simulink model "SecRwRtStFwdBkwdTrgtPosSelc"  (R2018b)
settings: Solver=FixedStepDiscrete  StartTime=0.0  StopTime=10.0  FixedStep=0.01  RelTol=1e-3
undefined symbols (not defined in the file or in its folder): KeSMSw4SAcsMd23SecRwRtStFrwdBkwdPos_Val, KeSMSw4SAcsMd23SecRwRtStFrwdBkwdPosMax_Val, KeSMSw4SAcsMd23SecRwRtStFrwdBkwdPosMin_Val, KeSMSw4SAcsMd24SecRwRtStFrwdBkwdPos_Val, KeSMSw4SAcsMd24SecRwRtStFrwdBkwdPosMax_Val, KeSMSw4SAcsMd24SecRwRtStFrwdBkwdPosMin_Val, KeSMSw4SAcsMd25SecRwRtStFrwdBkwdPos_Val, KeSMSw4SAcsMd25SecRwRtStFrwdBkwdPosMax_Val, KeSMSw4SAcsMd25SecRwRtStFrwdBkwdPosMin_Val, KeSMSw4SAcsMd26SecRwRtStFrwdBkwdPos_Val, KeSMSw4SAcsMd26SecRwRtStFrwdBkwdPosMax_Val, KeSMSw4SAcsMd26SecRwRtStFrwdBkwdPosMin_Val, KeSMSw4SLegrstOpenMdSecRwRtStFrwdBkwdPos_Val, KeSMSw4SLegrstOpenMdSecRwRtStFrwdBkwdPosMax_Val, KeSMSw4SLegrstOpenMdSecRwRtStFrwdBkwdPosMin_Val, KeSMSw4SLyingMDSecRwRtStFrwdBkwdPos_Val, KeSMSw4SLyingMDSecRwRtStFrwdBkwdPosMax_Val, KeSMSw4SLyingMDSecRwRtStFrwdBkwdPosMin_Val, KeSMSw4SVIPMDSecRwRtStFrwdBkwdPos_Val, KeSMSw4SVIPMDSecRwRtStFrwdBkwdPosMax_Val, KeSMSw4SVIPMDSecRwRtStFrwdBkwdPosMin_Val, KeSMSw6sAcsEntrySecRwRtStFrwdBkwdPos_Val, KeSMSw6sAcsEntrySecRwRtStFrwdBkwdPosMax_Val, KeSMSw6sAcsEntrySecRwRtStFrwdBkwdPosMin_Val, KeSMSw6sAcsExtSecRwRtStFrwdBkwdPos_Val, KeSMSw6sAcsExtSecRwRtStFrwdBkwdPosMax_Val, KeSMSw6sAcsExtSecRwRtStFrwdBkwdPosMin_Val, KeSMSw6sFamilyMdSecRwRtStFrwdBkwdPos_Val, KeSMSw6sFamilyMdSecRwRtStFrwdBkwdPosMax_Val, KeSMSw6sFamilyMdSecRwRtStFrwdBkwdPosMin_Val, KeSMSw6sFamilyRMdSecRwRtStFrwdBkwdPos_Val, KeSMSw6sFamilyRMdSecRwRtStFrwdBkwdPosMax_Val, KeSMSw6sFamilyRMdSecRwRtStFrwdBkwdPosMin_Val, KeSMSw6sVIPSecRwRtStFrwdBkwdPos_Val, KeSMSw6sVIPSecRwRtStFrwdBkwdPosMax_Val, KeSMSw6sVIPSecRwRtStFrwdBkwdPosMin_Val, KeSMSwAcsEntrySecRwRtStFrwdBkwdPos_Val, KeSMSwAcsEntrySecRwRtStFrwdBkwdPosMax_Val, KeSMSwAcsEntrySecRwRtStFrwdBkwdPosMin_Val, KeSMSwAcsExtSecRwRtStFrwdBkwdPos_Val, KeSMSwAcsExtSecRwRtStFrwdBkwdPosMax_Val, KeSMSwAcsExtSecRwRtStFrwdBkwdPosMin_Val, KeSMSwAcsMd8SecRwRtStFrwdBkwdPos_Val, KeSMSwAcsMd8SecRwRtStFrwdBkwdPosMax_Val, KeSMSwAcsMd8SecRwRtStFrwdBkwdPosMin_Val, KeSMSwAcsMd9SecRwRtStFrwdBkwdPos_Val, KeSMSwAcsMd9SecRwRtStFrwdBkwdPosMax_Val, KeSMSwAcsMd9SecRwRtStFrwdBkwdPosMin_Val, KeSMSwFamilyMdSecRwRtStFrwdBkwdPos_Val, KeSMSwFamilyMdSecRwRtStFrwdBkwdPosMax_Val, KeSMSwFamilyMdSecRwRtStFrwdBkwdPosMin_Val, KeSMSwFamilyRMdSecRwRtStFrwdBkwdPos_Val, KeSMSwFamilyRMdSecRwRtStFrwdBkwdPosMax_Val, KeSMSwFamilyRMdSecRwRtStFrwdBkwdPosMin_Val, KeSMSwVIPSecRwRtStFrwdBkwdPos_Val, KeSMSwVIPSecRwRtStFrwdBkwdPosMax_Val, KeSMSwVIPSecRwRtStFrwdBkwdPosMin_Val
libraries: TrgtPosSelcLib x16
settings Model: Creator=sn2xws  LastModifiedBy=sn2xws
settings Model: ModifiedHistory=|
  | 2023.8.1 V2.0.0 CR401790 增加模式21-26
  | Issue 566045 全躺，vip，腿托打开增加前后位置
  | 2024.7.9 V3.0.0 557模式流程V1.9
settings DataIOCC: SaveFormat=StructureWithTime
settings OptimizationCC: DefaultParameterBehavior=Inlined  EnhancedBackFolding=on  PassReuseOutputArgsAs=Individual arguments  ZeroExternalMemoryAtStartup=off  ZeroInternalMemoryAtStartup=off  OptimizeBlockOrder=speed  DifferentSizesBufferReuse=on  OptimizationCustomize=off
settings DebuggingCC: ParameterTunabilityLossMsg=error
settings ModelReferenceCC: ModelReferenceNumInstancesAllowed=Single
settings SFSimCC: MATLABDynamicMemAlloc=off
settings RTWCC: SystemTargetFile=autosar.tlc  GenCodeOnly=on  TemplateMakefile=ert_default_tmf  Description=AUTOSAR  GenerateReport=on  IncludeHyperlinkInReport=on  LaunchReport=on  GenerateTraceInfo=on  GenerateTraceReport=on  GenerateTraceReportSl=on  GenerateTraceReportSf=on  GenerateTraceReportEml=on
settings CodeAppCC: ForceParamTrailComments=on  IgnoreCustomStorageClasses=off  OperatorAnnotations=on  SimulinkDataObjDesc=on  SFDataObjDesc=on  InsertBlockDesc=on
settings STFCustomTargetCC: TargetLangStandard=C99 (ISO)  MultiwordLength=256  ParMdlRefBuildCompliant=on  CompOptLevelCompliant=on  IncludeMdlTerminateFcn=off  CombineOutputUpdateFcns=on  SuppressErrorStatus=on  ERTCustomFileBanners=on  SupportNonFinite=off  SupportComplex=off  SupportContinuousTime=off  SupportNonInlinedSFcns=off  RemoveResetFunc=on  MATLABClassNameForMDSCustomization=Simulink.SoftwareTarget.ERTCustomization  AutosarCompliant=on  UseToolchainInfoCompliant=on  LookupTableObjectStructAxisOrder=2,1,3,4,...  LUTObjectStructOrderEvenSpacing=Size,Table,Breakpoints  SystemTargetFile=autosar.tlc
settings ERTTargetCC: TargetLangStandard=C99 (ISO)  ConcurrentExecutionCompliant=off  IncludeMdlTerminateFcn=off  SuppressErrorStatus=on  SupportNonFinite=off  SupportComplex=off  ModelStepFunctionPrototypeControlCompliant=off  CPPClassGenCompliant=off  AutosarCompliant=on  LookupTableObjectStructAxisOrder=2,1,3,4,...  LUTObjectStructOrderEvenSpacing=Size,Table,Breakpoints  InlinedParameterPlacement=NonHierarchical  ERTCustomFileTemplate=example_file_process.tlc  ERTFilePackagingFormat=Compact

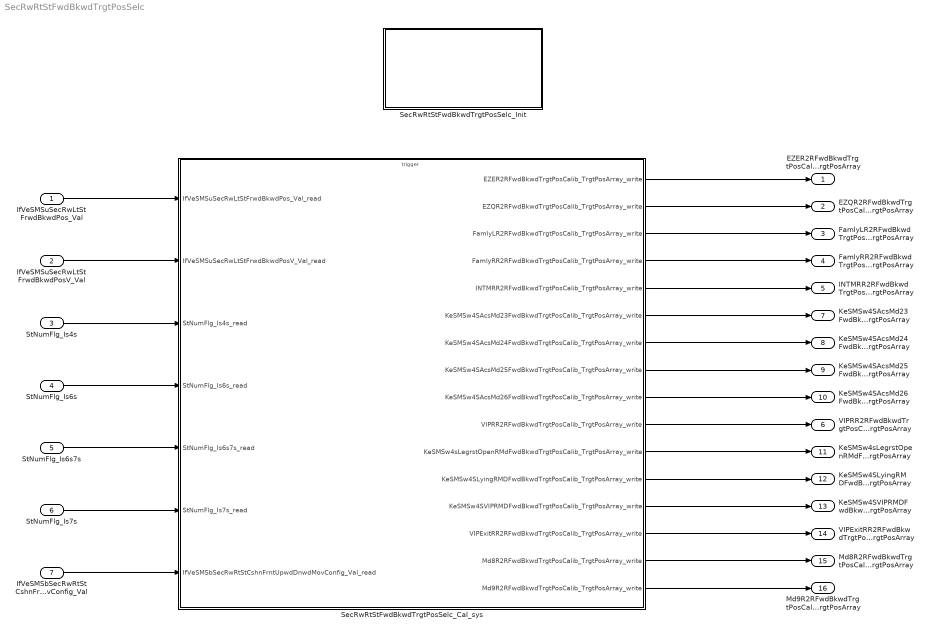
== system SecRwRtStFwdBkwdTrgtPosSelc ==
  IfVeSMSuSecRwLtStFrwdBkwdPos_Val : Inport  OutDataTypeStr=uint16  PortDimensions=1
  IfVeSMSuSecRwLtStFrwdBkwdPosV_Val : Inport  Port=2  OutDataTypeStr=boolean  PortDimensions=1
  StNumFlg_Is4s : Inport  Port=3  OutDataTypeStr=boolean  PortDimensions=1
  StNumFlg_Is6s : Inport  Port=4  OutDataTypeStr=boolean  PortDimensions=1
  StNumFlg_Is6s7s : Inport  Port=5  OutDataTypeStr=boolean  PortDimensions=1
  StNumFlg_Is7s : Inport  Port=6  OutDataTypeStr=boolean  PortDimensions=1
  IfVeSMSbSecRwRtStCshnFrntUpwdDnwdMovConfig_Val : Inport  Port=7  OutDataTypeStr=boolean  PortDimensions=1
  SecRwRtStFwdBkwdTrgtPosSelc_Cal_sys : Subsystem
  SecRwRtStFwdBkwdTrgtPosSelc_Init : Subsystem
  EZER2RFwdBkwdTrgtPosCalib_TrgtPosArray : Outport  Description=|  OutDataTypeStr=uint16  PortDimensions=3
      | 0:Pos
      | 1:Max
      | 2:Min
  EZQR2RFwdBkwdTrgtPosCalib_TrgtPosArray : Outport  Description=|  Port=2  OutDataTypeStr=uint16  PortDimensions=3
      | 0:Pos
      | 1:Max
      | 2:Min
  FamlyLR2RFwdBkwdTrgtPosCalib_TrgtPosArray : Outport  Description=|  Port=3  OutDataTypeStr=uint16  PortDimensions=3
      | 0:Pos
      | 1:Max
      | 2:Min
  FamlyRR2RFwdBkwdTrgtPosCalib_TrgtPosArray : Outport  Description=|  Port=4  OutDataTypeStr=uint16  PortDimensions=3
      | 0:Pos
      | 1:Max
      | 2:Min
  INTMRR2RFwdBkwdTrgtPosCalib_TrgtPosArray : Outport  Description=|  Port=5  OutDataTypeStr=uint16  PortDimensions=3
      | 0:Pos
      | 1:Max
      | 2:Min
  VIPRR2RFwdBkwdTrgtPosCalib_TrgtPosArray : Outport  Description=|  Port=6  OutDataTypeStr=uint16  PortDimensions=3
      | 0:Pos
      | 1:Max
      | 2:Min
  KeSMSw4SAcsMd23FwdBkwdTrgtPosCalib_TrgtPosArray : Outport  Description=|  Port=7  OutDataTypeStr=uint16  PortDimensions=3
      | 0:Pos
      | 1:Max
      | 2:Min
  KeSMSw4SAcsMd24FwdBkwdTrgtPosCalib_TrgtPosArray : Outport  Description=|  Port=8  OutDataTypeStr=uint16  PortDimensions=3
      | 0:Pos
      | 1:Max
      | 2:Min
  KeSMSw4SAcsMd25FwdBkwdTrgtPosCalib_TrgtPosArray : Outport  Description=|  Port=9  OutDataTypeStr=uint16  PortDimensions=3
      | 0:Pos
      | 1:Max
      | 2:Min
  KeSMSw4SAcsMd26FwdBkwdTrgtPosCalib_TrgtPosArray : Outport  Description=|  Port=10  OutDataTypeStr=uint16  PortDimensions=3
      | 0:Pos
      | 1:Max
      | 2:Min
  KeSMSw4sLegrstOpenRMdFwdBkwdTrgtPosCalib_TrgtPosArray : Outport  Description=|  Port=11  OutDataTypeStr=uint16  PortDimensions=3
      | 0:Pos
      | 1:Max
      | 2:Min
  KeSMSw4SLyingRMDFwdBkwdTrgtPosCalib_TrgtPosArray : Outport  Description=|  Port=12  OutDataTypeStr=uint16  PortDimensions=3
      | 0:Pos
      | 1:Max
      | 2:Min
  KeSMSw4SVIPRMDFwdBkwdTrgtPosCalib_TrgtPosArray : Outport  Description=|  Port=13  OutDataTypeStr=uint16  PortDimensions=3
      | 0:Pos
      | 1:Max
      | 2:Min
  VIPExitRR2RFwdBkwdTrgtPosCalib_TrgtPosArray : Outport  Description=|  Port=14  OutDataTypeStr=uint16  PortDimensions=3
      | 0:Pos
      | 1:Max
      | 2:Min
  Md8R2RFwdBkwdTrgtPosCalib_TrgtPosArray : Outport  Description=|  Port=15  OutDataTypeStr=uint16  PortDimensions=3
      | 0:Pos
      | 1:Max
      | 2:Min
  Md9R2RFwdBkwdTrgtPosCalib_TrgtPosArray : Outport  Description=|  Port=16  OutDataTypeStr=uint16  PortDimensions=3
      | 0:Pos
      | 1:Max
      | 2:Min
  wires:
  IfVeSMSuSecRwLtStFrwdBkwdPos_Val/1 -> SecRwRtStFwdBkwdTrgtPosSelc_Cal_sys/1(IfVeSMSuSecRwLtStFrwdBkwdPos_Val_read)
  IfVeSMSuSecRwLtStFrwdBkwdPosV_Val/1 -> SecRwRtStFwdBkwdTrgtPosSelc_Cal_sys/2(IfVeSMSuSecRwLtStFrwdBkwdPosV_Val_read)
  StNumFlg_Is4s/1 -> SecRwRtStFwdBkwdTrgtPosSelc_Cal_sys/3(StNumFlg_Is4s_read)
  StNumFlg_Is6s/1 -> SecRwRtStFwdBkwdTrgtPosSelc_Cal_sys/4(StNumFlg_Is6s_read)
  StNumFlg_Is6s7s/1 -> SecRwRtStFwdBkwdTrgtPosSelc_Cal_sys/5(StNumFlg_Is6s7s_read)
  StNumFlg_Is7s/1 -> SecRwRtStFwdBkwdTrgtPosSelc_Cal_sys/6(StNumFlg_Is7s_read)
  SecRwRtStFwdBkwdTrgtPosSelc_Cal_sys/1(EZER2RFwdBkwdTrgtPosCalib_TrgtPosArray_write) -> EZER2RFwdBkwdTrgtPosCalib_TrgtPosArray/1
  SecRwRtStFwdBkwdTrgtPosSelc_Cal_sys/2(EZQR2RFwdBkwdTrgtPosCalib_TrgtPosArray_write) -> EZQR2RFwdBkwdTrgtPosCalib_TrgtPosArray/1
  SecRwRtStFwdBkwdTrgtPosSelc_Cal_sys/3(FamlyLR2RFwdBkwdTrgtPosCalib_TrgtPosArray_write) -> FamlyLR2RFwdBkwdTrgtPosCalib_TrgtPosArray/1
  SecRwRtStFwdBkwdTrgtPosSelc_Cal_sys/4(FamlyRR2RFwdBkwdTrgtPosCalib_TrgtPosArray_write) -> FamlyRR2RFwdBkwdTrgtPosCalib_TrgtPosArray/1
  SecRwRtStFwdBkwdTrgtPosSelc_Cal_sys/5(INTMRR2RFwdBkwdTrgtPosCalib_TrgtPosArray_write) -> INTMRR2RFwdBkwdTrgtPosCalib_TrgtPosArray/1
  SecRwRtStFwdBkwdTrgtPosSelc_Cal_sys/10(VIPRR2RFwdBkwdTrgtPosCalib_TrgtPosArray_write) -> VIPRR2RFwdBkwdTrgtPosCalib_TrgtPosArray/1
  SecRwRtStFwdBkwdTrgtPosSelc_Cal_sys/6(KeSMSw4SAcsMd23FwdBkwdTrgtPosCalib_TrgtPosArray_write) -> KeSMSw4SAcsMd23FwdBkwdTrgtPosCalib_TrgtPosArray/1
  SecRwRtStFwdBkwdTrgtPosSelc_Cal_sys/7(KeSMSw4SAcsMd24FwdBkwdTrgtPosCalib_TrgtPosArray_write) -> KeSMSw4SAcsMd24FwdBkwdTrgtPosCalib_TrgtPosArray/1
  SecRwRtStFwdBkwdTrgtPosSelc_Cal_sys/8(KeSMSw4SAcsMd25FwdBkwdTrgtPosCalib_TrgtPosArray_write) -> KeSMSw4SAcsMd25FwdBkwdTrgtPosCalib_TrgtPosArray/1
  SecRwRtStFwdBkwdTrgtPosSelc_Cal_sys/9(KeSMSw4SAcsMd26FwdBkwdTrgtPosCalib_TrgtPosArray_write) -> KeSMSw4SAcsMd26FwdBkwdTrgtPosCalib_TrgtPosArray/1
  SecRwRtStFwdBkwdTrgtPosSelc_Cal_sys/11(KeSMSw4sLegrstOpenRMdFwdBkwdTrgtPosCalib_TrgtPosArray_write) -> KeSMSw4sLegrstOpenRMdFwdBkwdTrgtPosCalib_TrgtPosArray/1
  SecRwRtStFwdBkwdTrgtPosSelc_Cal_sys/12(KeSMSw4SLyingRMDFwdBkwdTrgtPosCalib_TrgtPosArray_write) -> KeSMSw4SLyingRMDFwdBkwdTrgtPosCalib_TrgtPosArray/1
  SecRwRtStFwdBkwdTrgtPosSelc_Cal_sys/13(KeSMSw4SVIPRMDFwdBkwdTrgtPosCalib_TrgtPosArray_write) -> KeSMSw4SVIPRMDFwdBkwdTrgtPosCalib_TrgtPosArray/1
  IfVeSMSbSecRwRtStCshnFrntUpwdDnwdMovConfig_Val/1 -> SecRwRtStFwdBkwdTrgtPosSelc_Cal_sys/7(IfVeSMSbSecRwRtStCshnFrntUpwdDnwdMovConfig_Val_read)
  SecRwRtStFwdBkwdTrgtPosSelc_Cal_sys/14(VIPExitRR2RFwdBkwdTrgtPosCalib_TrgtPosArray_write) -> VIPExitRR2RFwdBkwdTrgtPosCalib_TrgtPosArray/1
  SecRwRtStFwdBkwdTrgtPosSelc_Cal_sys/15(Md8R2RFwdBkwdTrgtPosCalib_TrgtPosArray_write) -> Md8R2RFwdBkwdTrgtPosCalib_TrgtPosArray/1
  SecRwRtStFwdBkwdTrgtPosSelc_Cal_sys/16(Md9R2RFwdBkwdTrgtPosCalib_TrgtPosArray_write) -> Md9R2RFwdBkwdTrgtPosCalib_TrgtPosArray/1

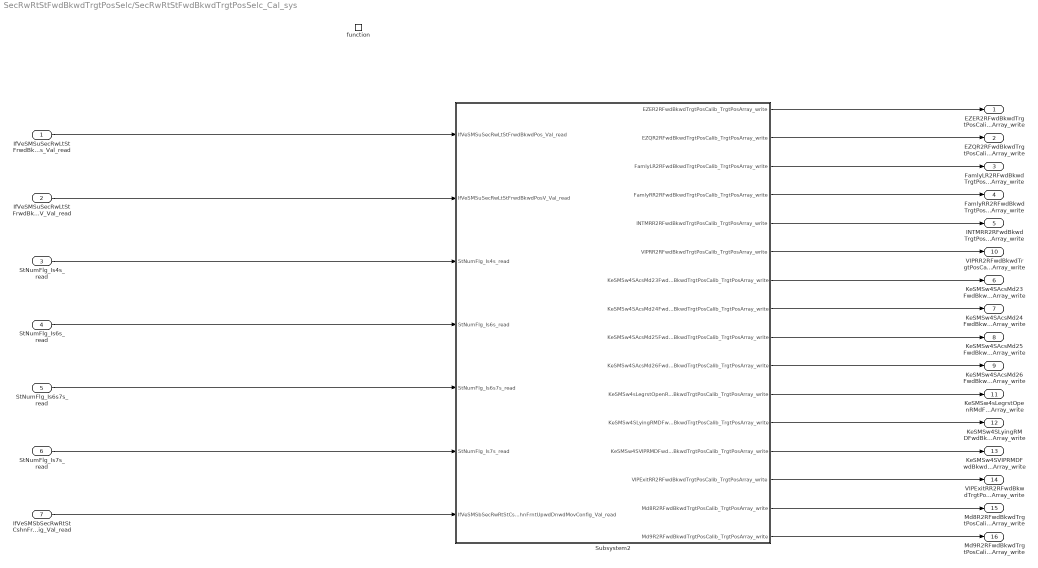
== system SecRwRtStFwdBkwdTrgtPosSelc/SecRwRtStFwdBkwdTrgtPosSelc_Cal_sys ==
  IfVeSMSuSecRwLtStFrwdBkwdPos_Val_read : Inport
  IfVeSMSuSecRwLtStFrwdBkwdPosV_Val_read : Inport  Port=2
  StNumFlg_Is4s_read : Inport  Port=3
  StNumFlg_Is6s_read : Inport  Port=4
  StNumFlg_Is6s7s_read : Inport  Port=5
  StNumFlg_Is7s_read : Inport  Port=6
  IfVeSMSbSecRwRtStCshnFrntUpwdDnwdMovConfig_Val_read : Inport  Port=7
  function : TriggerPort  TriggerType=function-call  IsSimulinkFunction=on  FunctionName=SecRwRtStFwdBkwdTrgtPosSelc_Cal  VariantControl=(inherit)
  Subsystem2 : Subsystem
  EZER2RFwdBkwdTrgtPosCalib_TrgtPosArray_write : Outport
      settings: EnsureOutportIsVirtual=on
  EZQR2RFwdBkwdTrgtPosCalib_TrgtPosArray_write : Outport  Port=2
      settings: EnsureOutportIsVirtual=on
  FamlyLR2RFwdBkwdTrgtPosCalib_TrgtPosArray_write : Outport  Port=3
      settings: EnsureOutportIsVirtual=on
  FamlyRR2RFwdBkwdTrgtPosCalib_TrgtPosArray_write : Outport  Port=4
      settings: EnsureOutportIsVirtual=on
  INTMRR2RFwdBkwdTrgtPosCalib_TrgtPosArray_write : Outport  Port=5
      settings: EnsureOutportIsVirtual=on
  KeSMSw4SAcsMd23FwdBkwdTrgtPosCalib_TrgtPosArray_write : Outport  Port=6
      settings: EnsureOutportIsVirtual=on
  KeSMSw4SAcsMd24FwdBkwdTrgtPosCalib_TrgtPosArray_write : Outport  Port=7
      settings: EnsureOutportIsVirtual=on
  KeSMSw4SAcsMd25FwdBkwdTrgtPosCalib_TrgtPosArray_write : Outport  Port=8
      settings: EnsureOutportIsVirtual=on
  KeSMSw4SAcsMd26FwdBkwdTrgtPosCalib_TrgtPosArray_write : Outport  Port=9
      settings: EnsureOutportIsVirtual=on
  VIPRR2RFwdBkwdTrgtPosCalib_TrgtPosArray_write : Outport  Port=10
      settings: EnsureOutportIsVirtual=on
  KeSMSw4sLegrstOpenRMdFwdBkwdTrgtPosCalib_TrgtPosArray_write : Outport  Port=11
      settings: EnsureOutportIsVirtual=on
  KeSMSw4SLyingRMDFwdBkwdTrgtPosCalib_TrgtPosArray_write : Outport  Port=12
      settings: EnsureOutportIsVirtual=on
  KeSMSw4SVIPRMDFwdBkwdTrgtPosCalib_TrgtPosArray_write : Outport  Port=13
      settings: EnsureOutportIsVirtual=on
  VIPExitRR2RFwdBkwdTrgtPosCalib_TrgtPosArray_write : Outport  Port=14
      settings: EnsureOutportIsVirtual=on
  Md8R2RFwdBkwdTrgtPosCalib_TrgtPosArray_write : Outport  Port=15
      settings: EnsureOutportIsVirtual=on
  Md9R2RFwdBkwdTrgtPosCalib_TrgtPosArray_write : Outport  Port=16
      settings: EnsureOutportIsVirtual=on
  wires:
  Subsystem2/6(VIPRR2RFwdBkwdTrgtPosCalib_TrgtPosArray_write) -> VIPRR2RFwdBkwdTrgtPosCalib_TrgtPosArray_write/1
  Subsystem2/3(FamlyLR2RFwdBkwdTrgtPosCalib_TrgtPosArray_write) -> FamlyLR2RFwdBkwdTrgtPosCalib_TrgtPosArray_write/1
  Subsystem2/4(FamlyRR2RFwdBkwdTrgtPosCalib_TrgtPosArray_write) -> FamlyRR2RFwdBkwdTrgtPosCalib_TrgtPosArray_write/1
  Subsystem2/2(EZQR2RFwdBkwdTrgtPosCalib_TrgtPosArray_write) -> EZQR2RFwdBkwdTrgtPosCalib_TrgtPosArray_write/1
  Subsystem2/5(INTMRR2RFwdBkwdTrgtPosCalib_TrgtPosArray_write) -> INTMRR2RFwdBkwdTrgtPosCalib_TrgtPosArray_write/1
  Subsystem2/7(KeSMSw4SAcsMd23FwdBkwdTrgtPosCalib_TrgtPosArray_write) -> KeSMSw4SAcsMd23FwdBkwdTrgtPosCalib_TrgtPosArray_write/1
  Subsystem2/1(EZER2RFwdBkwdTrgtPosCalib_TrgtPosArray_write) -> EZER2RFwdBkwdTrgtPosCalib_TrgtPosArray_write/1
  Subsystem2/8(KeSMSw4SAcsMd24FwdBkwdTrgtPosCalib_TrgtPosArray_write) -> KeSMSw4SAcsMd24FwdBkwdTrgtPosCalib_TrgtPosArray_write/1
  Subsystem2/9(KeSMSw4SAcsMd25FwdBkwdTrgtPosCalib_TrgtPosArray_write) -> KeSMSw4SAcsMd25FwdBkwdTrgtPosCalib_TrgtPosArray_write/1
  Subsystem2/10(KeSMSw4SAcsMd26FwdBkwdTrgtPosCalib_TrgtPosArray_write) -> KeSMSw4SAcsMd26FwdBkwdTrgtPosCalib_TrgtPosArray_write/1
  IfVeSMSuSecRwLtStFrwdBkwdPos_Val_read/1 -> Subsystem2/1(IfVeSMSuSecRwLtStFrwdBkwdPos_Val_read)
  IfVeSMSuSecRwLtStFrwdBkwdPosV_Val_read/1 -> Subsystem2/2(IfVeSMSuSecRwLtStFrwdBkwdPosV_Val_read)
  StNumFlg_Is4s_read/1 -> Subsystem2/3(StNumFlg_Is4s_read)
  StNumFlg_Is6s_read/1 -> Subsystem2/4(StNumFlg_Is6s_read)
  StNumFlg_Is6s7s_read/1 -> Subsystem2/5(StNumFlg_Is6s7s_read)
  StNumFlg_Is7s_read/1 -> Subsystem2/6(StNumFlg_Is7s_read)
  Subsystem2/11(KeSMSw4sLegrstOpenRMdFwdBkwdTrgtPosCalib_TrgtPosArray_write) -> KeSMSw4sLegrstOpenRMdFwdBkwdTrgtPosCalib_TrgtPosArray_write/1
  Subsystem2/12(KeSMSw4SLyingRMDFwdBkwdTrgtPosCalib_TrgtPosArray_write) -> KeSMSw4SLyingRMDFwdBkwdTrgtPosCalib_TrgtPosArray_write/1
  Subsystem2/13(KeSMSw4SVIPRMDFwdBkwdTrgtPosCalib_TrgtPosArray_write) -> KeSMSw4SVIPRMDFwdBkwdTrgtPosCalib_TrgtPosArray_write/1
  Subsystem2/14(VIPExitRR2RFwdBkwdTrgtPosCalib_TrgtPosArray_write) -> VIPExitRR2RFwdBkwdTrgtPosCalib_TrgtPosArray_write/1
  IfVeSMSbSecRwRtStCshnFrntUpwdDnwdMovConfig_Val_read/1 -> Subsystem2/7(IfVeSMSbSecRwRtStCshnFrntUpwdDnwdMovConfig_Val_read)
  Subsystem2/15(Md8R2RFwdBkwdTrgtPosCalib_TrgtPosArray_write) -> Md8R2RFwdBkwdTrgtPosCalib_TrgtPosArray_write/1
  Subsystem2/16(Md9R2RFwdBkwdTrgtPosCalib_TrgtPosArray_write) -> Md9R2RFwdBkwdTrgtPosCalib_TrgtPosArray_write/1

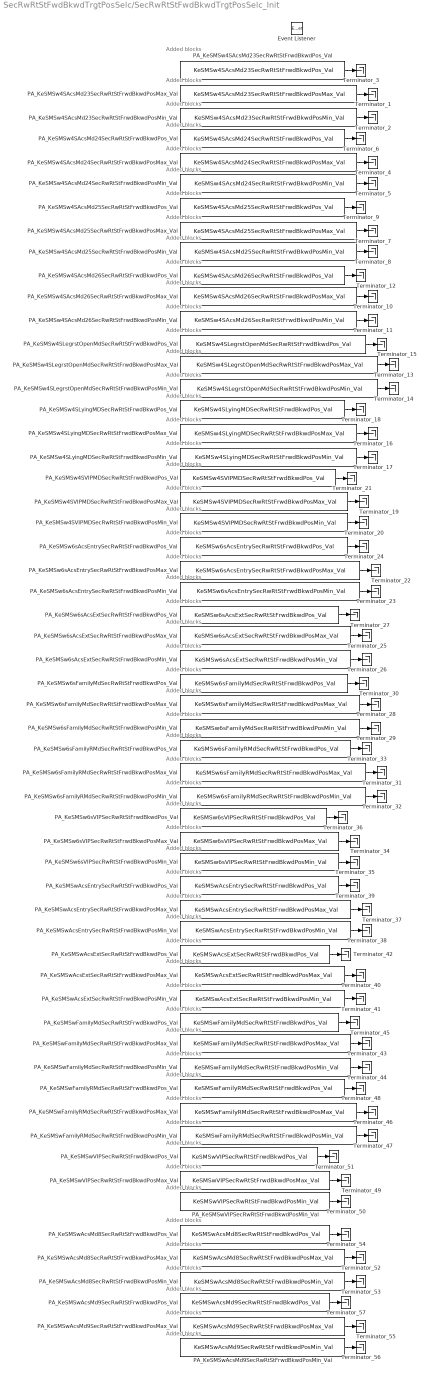
== system SecRwRtStFwdBkwdTrgtPosSelc/SecRwRtStFwdBkwdTrgtPosSelc_Init ==
  note: Added blocks
  note: Added blocks
  note: Added blocks
  note: Added blocks
  note: Added blocks
  note: Added blocks
  note: Added blocks
  note: Added blocks
  note: Added blocks
  note: Added blocks
  note: Added blocks
  note: Added blocks
  note: Added blocks
  note: Added blocks
  note: Added blocks
  note: Added blocks
  note: Added blocks
  note: Added blocks
  note: Added blocks
  note: Added blocks
  note: Added blocks
  note: Added blocks
  note: Added blocks
  note: Added blocks
  note: Added blocks
  note: Added blocks
  note: Added blocks
  note: Added blocks
  note: Added blocks
  note: Added blocks
  note: Added blocks
  note: Added blocks
  note: Added blocks
  note: Added blocks
  note: Added blocks
  note: Added blocks
  note: Added blocks
  note: Added blocks
  note: Added blocks
  note: Added blocks
  note: Added blocks
  note: Added blocks
  note: Added blocks
  note: Added blocks
  note: Added blocks
  note: Added blocks
  note: Added blocks
  note: Added blocks
  note: Added blocks
  note: Added blocks
  note: Added blocks
  note: Added blocks
  note: Added blocks
  note: Added blocks
  note: Added blocks
  note: Added blocks
  note: Added blocks
  Event Listener : EventListener  EventName=reset
  PA_KeSMSw4SAcsMd23SecRwRtStFrwdBkwdPosMax_Val : Constant  Value=KeSMSw4SAcsMd23SecRwRtStFrwdBkwdPosMax_Val
  PA_KeSMSw4SAcsMd23SecRwRtStFrwdBkwdPosMin_Val : Constant  Value=KeSMSw4SAcsMd23SecRwRtStFrwdBkwdPosMin_Val
  PA_KeSMSw4SAcsMd23SecRwRtStFrwdBkwdPos_Val : Constant  Value=KeSMSw4SAcsMd23SecRwRtStFrwdBkwdPos_Val
  PA_KeSMSw4SAcsMd24SecRwRtStFrwdBkwdPosMax_Val : Constant  Value=KeSMSw4SAcsMd24SecRwRtStFrwdBkwdPosMax_Val
  PA_KeSMSw4SAcsMd24SecRwRtStFrwdBkwdPosMin_Val : Constant  Value=KeSMSw4SAcsMd24SecRwRtStFrwdBkwdPosMin_Val
  PA_KeSMSw4SAcsMd24SecRwRtStFrwdBkwdPos_Val : Constant  Value=KeSMSw4SAcsMd24SecRwRtStFrwdBkwdPos_Val
  PA_KeSMSw4SAcsMd25SecRwRtStFrwdBkwdPosMax_Val : Constant  Value=KeSMSw4SAcsMd25SecRwRtStFrwdBkwdPosMax_Val
  PA_KeSMSw4SAcsMd25SecRwRtStFrwdBkwdPosMin_Val : Constant  Value=KeSMSw4SAcsMd25SecRwRtStFrwdBkwdPosMin_Val
  PA_KeSMSw4SAcsMd25SecRwRtStFrwdBkwdPos_Val : Constant  Value=KeSMSw4SAcsMd25SecRwRtStFrwdBkwdPos_Val
  PA_KeSMSw4SAcsMd26SecRwRtStFrwdBkwdPosMax_Val : Constant  Value=KeSMSw4SAcsMd26SecRwRtStFrwdBkwdPosMax_Val
  PA_KeSMSw4SAcsMd26SecRwRtStFrwdBkwdPosMin_Val : Constant  Value=KeSMSw4SAcsMd26SecRwRtStFrwdBkwdPosMin_Val
  PA_KeSMSw4SAcsMd26SecRwRtStFrwdBkwdPos_Val : Constant  Value=KeSMSw4SAcsMd26SecRwRtStFrwdBkwdPos_Val
  PA_KeSMSw4SLegrstOpenMdSecRwRtStFrwdBkwdPosMax_Val : Constant  Value=KeSMSw4SLegrstOpenMdSecRwRtStFrwdBkwdPosMax_Val
  PA_KeSMSw4SLegrstOpenMdSecRwRtStFrwdBkwdPosMin_Val : Constant  Value=KeSMSw4SLegrstOpenMdSecRwRtStFrwdBkwdPosMin_Val
  PA_KeSMSw4SLegrstOpenMdSecRwRtStFrwdBkwdPos_Val : Constant  Value=KeSMSw4SLegrstOpenMdSecRwRtStFrwdBkwdPos_Val
  PA_KeSMSw4SLyingMDSecRwRtStFrwdBkwdPosMax_Val : Constant  Value=KeSMSw4SLyingMDSecRwRtStFrwdBkwdPosMax_Val
  PA_KeSMSw4SLyingMDSecRwRtStFrwdBkwdPosMin_Val : Constant  Value=KeSMSw4SLyingMDSecRwRtStFrwdBkwdPosMin_Val
  PA_KeSMSw4SLyingMDSecRwRtStFrwdBkwdPos_Val : Constant  Value=KeSMSw4SLyingMDSecRwRtStFrwdBkwdPos_Val
  PA_KeSMSw4SVIPMDSecRwRtStFrwdBkwdPosMax_Val : Constant  Value=KeSMSw4SVIPMDSecRwRtStFrwdBkwdPosMax_Val
  PA_KeSMSw4SVIPMDSecRwRtStFrwdBkwdPosMin_Val : Constant  Value=KeSMSw4SVIPMDSecRwRtStFrwdBkwdPosMin_Val
  PA_KeSMSw4SVIPMDSecRwRtStFrwdBkwdPos_Val : Constant  Value=KeSMSw4SVIPMDSecRwRtStFrwdBkwdPos_Val
  PA_KeSMSw6sAcsEntrySecRwRtStFrwdBkwdPosMax_Val : Constant  Value=KeSMSw6sAcsEntrySecRwRtStFrwdBkwdPosMax_Val
  PA_KeSMSw6sAcsEntrySecRwRtStFrwdBkwdPosMin_Val : Constant  Value=KeSMSw6sAcsEntrySecRwRtStFrwdBkwdPosMin_Val
  PA_KeSMSw6sAcsEntrySecRwRtStFrwdBkwdPos_Val : Constant  Value=KeSMSw6sAcsEntrySecRwRtStFrwdBkwdPos_Val
  PA_KeSMSw6sAcsExtSecRwRtStFrwdBkwdPosMax_Val : Constant  Value=KeSMSw6sAcsExtSecRwRtStFrwdBkwdPosMax_Val
  PA_KeSMSw6sAcsExtSecRwRtStFrwdBkwdPosMin_Val : Constant  Value=KeSMSw6sAcsExtSecRwRtStFrwdBkwdPosMin_Val
  PA_KeSMSw6sAcsExtSecRwRtStFrwdBkwdPos_Val : Constant  Value=KeSMSw6sAcsExtSecRwRtStFrwdBkwdPos_Val
  PA_KeSMSw6sFamilyMdSecRwRtStFrwdBkwdPosMax_Val : Constant  Value=KeSMSw6sFamilyMdSecRwRtStFrwdBkwdPosMax_Val
  PA_KeSMSw6sFamilyMdSecRwRtStFrwdBkwdPosMin_Val : Constant  Value=KeSMSw6sFamilyMdSecRwRtStFrwdBkwdPosMin_Val
  PA_KeSMSw6sFamilyMdSecRwRtStFrwdBkwdPos_Val : Constant  Value=KeSMSw6sFamilyMdSecRwRtStFrwdBkwdPos_Val
  PA_KeSMSw6sFamilyRMdSecRwRtStFrwdBkwdPosMax_Val : Constant  Value=KeSMSw6sFamilyRMdSecRwRtStFrwdBkwdPosMax_Val
  PA_KeSMSw6sFamilyRMdSecRwRtStFrwdBkwdPosMin_Val : Constant  Value=KeSMSw6sFamilyRMdSecRwRtStFrwdBkwdPosMin_Val
  PA_KeSMSw6sFamilyRMdSecRwRtStFrwdBkwdPos_Val : Constant  Value=KeSMSw6sFamilyRMdSecRwRtStFrwdBkwdPos_Val
  PA_KeSMSw6sVIPSecRwRtStFrwdBkwdPosMax_Val : Constant  Value=KeSMSw6sVIPSecRwRtStFrwdBkwdPosMax_Val
  PA_KeSMSw6sVIPSecRwRtStFrwdBkwdPosMin_Val : Constant  Value=KeSMSw6sVIPSecRwRtStFrwdBkwdPosMin_Val
  PA_KeSMSw6sVIPSecRwRtStFrwdBkwdPos_Val : Constant  Value=KeSMSw6sVIPSecRwRtStFrwdBkwdPos_Val
  PA_KeSMSwAcsEntrySecRwRtStFrwdBkwdPosMax_Val : Constant  Value=KeSMSwAcsEntrySecRwRtStFrwdBkwdPosMax_Val
  PA_KeSMSwAcsEntrySecRwRtStFrwdBkwdPosMin_Val : Constant  Value=KeSMSwAcsEntrySecRwRtStFrwdBkwdPosMin_Val
  PA_KeSMSwAcsEntrySecRwRtStFrwdBkwdPos_Val : Constant  Value=KeSMSwAcsEntrySecRwRtStFrwdBkwdPos_Val
  PA_KeSMSwAcsExtSecRwRtStFrwdBkwdPosMax_Val : Constant  Value=KeSMSwAcsExtSecRwRtStFrwdBkwdPosMax_Val
  PA_KeSMSwAcsExtSecRwRtStFrwdBkwdPosMin_Val : Constant  Value=KeSMSwAcsExtSecRwRtStFrwdBkwdPosMin_Val
  PA_KeSMSwAcsExtSecRwRtStFrwdBkwdPos_Val : Constant  Value=KeSMSwAcsExtSecRwRtStFrwdBkwdPos_Val
  PA_KeSMSwAcsMd8SecRwRtStFrwdBkwdPosMax_Val : Constant  Value=KeSMSwAcsMd8SecRwRtStFrwdBkwdPosMax_Val
  PA_KeSMSwAcsMd8SecRwRtStFrwdBkwdPosMin_Val : Constant  Value=KeSMSwAcsMd8SecRwRtStFrwdBkwdPosMin_Val
  PA_KeSMSwAcsMd8SecRwRtStFrwdBkwdPos_Val : Constant  Value=KeSMSwAcsMd8SecRwRtStFrwdBkwdPos_Val
  PA_KeSMSwAcsMd9SecRwRtStFrwdBkwdPosMax_Val : Constant  Value=KeSMSwAcsMd9SecRwRtStFrwdBkwdPosMax_Val
  PA_KeSMSwAcsMd9SecRwRtStFrwdBkwdPosMin_Val : Constant  Value=KeSMSwAcsMd9SecRwRtStFrwdBkwdPosMin_Val
  PA_KeSMSwAcsMd9SecRwRtStFrwdBkwdPos_Val : Constant  Value=KeSMSwAcsMd9SecRwRtStFrwdBkwdPos_Val
  PA_KeSMSwFamilyMdSecRwRtStFrwdBkwdPosMax_Val : Constant  Value=KeSMSwFamilyMdSecRwRtStFrwdBkwdPosMax_Val
  PA_KeSMSwFamilyMdSecRwRtStFrwdBkwdPosMin_Val : Constant  Value=KeSMSwFamilyMdSecRwRtStFrwdBkwdPosMin_Val
  PA_KeSMSwFamilyMdSecRwRtStFrwdBkwdPos_Val : Constant  Value=KeSMSwFamilyMdSecRwRtStFrwdBkwdPos_Val
  PA_KeSMSwFamilyRMdSecRwRtStFrwdBkwdPosMax_Val : Constant  Value=KeSMSwFamilyRMdSecRwRtStFrwdBkwdPosMax_Val
  PA_KeSMSwFamilyRMdSecRwRtStFrwdBkwdPosMin_Val : Constant  Value=KeSMSwFamilyRMdSecRwRtStFrwdBkwdPosMin_Val
  PA_KeSMSwFamilyRMdSecRwRtStFrwdBkwdPos_Val : Constant  Value=KeSMSwFamilyRMdSecRwRtStFrwdBkwdPos_Val
  PA_KeSMSwVIPSecRwRtStFrwdBkwdPosMax_Val : Constant  Value=KeSMSwVIPSecRwRtStFrwdBkwdPosMax_Val
  PA_KeSMSwVIPSecRwRtStFrwdBkwdPosMin_Val : Constant  Value=KeSMSwVIPSecRwRtStFrwdBkwdPosMin_Val
  PA_KeSMSwVIPSecRwRtStFrwdBkwdPos_Val : Constant  Value=KeSMSwVIPSecRwRtStFrwdBkwdPos_Val
  Terminator_{1..57} (57 alike) : Terminator
  wires:
  PA_KeSMSw4SAcsMd23SecRwRtStFrwdBkwdPosMax_Val/1 -> Terminator_1/1
  PA_KeSMSw4SAcsMd23SecRwRtStFrwdBkwdPosMin_Val/1 -> Terminator_2/1
  PA_KeSMSw4SAcsMd23SecRwRtStFrwdBkwdPos_Val/1 -> Terminator_3/1
  PA_KeSMSw4SAcsMd24SecRwRtStFrwdBkwdPosMax_Val/1 -> Terminator_4/1
  PA_KeSMSw4SAcsMd24SecRwRtStFrwdBkwdPosMin_Val/1 -> Terminator_5/1
  PA_KeSMSw4SAcsMd24SecRwRtStFrwdBkwdPos_Val/1 -> Terminator_6/1
  PA_KeSMSw4SAcsMd25SecRwRtStFrwdBkwdPosMax_Val/1 -> Terminator_7/1
  PA_KeSMSw4SAcsMd25SecRwRtStFrwdBkwdPosMin_Val/1 -> Terminator_8/1
  PA_KeSMSw4SAcsMd25SecRwRtStFrwdBkwdPos_Val/1 -> Terminator_9/1
  PA_KeSMSw4SAcsMd26SecRwRtStFrwdBkwdPosMax_Val/1 -> Terminator_10/1
  PA_KeSMSw4SAcsMd26SecRwRtStFrwdBkwdPosMin_Val/1 -> Terminator_11/1
  PA_KeSMSw4SAcsMd26SecRwRtStFrwdBkwdPos_Val/1 -> Terminator_12/1
  PA_KeSMSw4SLegrstOpenMdSecRwRtStFrwdBkwdPosMax_Val/1 -> Terminator_13/1
  PA_KeSMSw4SLegrstOpenMdSecRwRtStFrwdBkwdPosMin_Val/1 -> Terminator_14/1
  PA_KeSMSw4SLegrstOpenMdSecRwRtStFrwdBkwdPos_Val/1 -> Terminator_15/1
  PA_KeSMSw4SLyingMDSecRwRtStFrwdBkwdPosMax_Val/1 -> Terminator_16/1
  PA_KeSMSw4SLyingMDSecRwRtStFrwdBkwdPosMin_Val/1 -> Terminator_17/1
  PA_KeSMSw4SLyingMDSecRwRtStFrwdBkwdPos_Val/1 -> Terminator_18/1
  PA_KeSMSw4SVIPMDSecRwRtStFrwdBkwdPosMax_Val/1 -> Terminator_19/1
  PA_KeSMSw4SVIPMDSecRwRtStFrwdBkwdPosMin_Val/1 -> Terminator_20/1
  PA_KeSMSw4SVIPMDSecRwRtStFrwdBkwdPos_Val/1 -> Terminator_21/1
  PA_KeSMSw6sAcsEntrySecRwRtStFrwdBkwdPosMax_Val/1 -> Terminator_22/1
  PA_KeSMSw6sAcsEntrySecRwRtStFrwdBkwdPosMin_Val/1 -> Terminator_23/1
  PA_KeSMSw6sAcsEntrySecRwRtStFrwdBkwdPos_Val/1 -> Terminator_24/1
  PA_KeSMSw6sAcsExtSecRwRtStFrwdBkwdPosMax_Val/1 -> Terminator_25/1
  PA_KeSMSw6sAcsExtSecRwRtStFrwdBkwdPosMin_Val/1 -> Terminator_26/1
  PA_KeSMSw6sAcsExtSecRwRtStFrwdBkwdPos_Val/1 -> Terminator_27/1
  PA_KeSMSw6sFamilyMdSecRwRtStFrwdBkwdPosMax_Val/1 -> Terminator_28/1
  PA_KeSMSw6sFamilyMdSecRwRtStFrwdBkwdPosMin_Val/1 -> Terminator_29/1
  PA_KeSMSw6sFamilyMdSecRwRtStFrwdBkwdPos_Val/1 -> Terminator_30/1
  PA_KeSMSw6sFamilyRMdSecRwRtStFrwdBkwdPosMax_Val/1 -> Terminator_31/1
  PA_KeSMSw6sFamilyRMdSecRwRtStFrwdBkwdPosMin_Val/1 -> Terminator_32/1
  PA_KeSMSw6sFamilyRMdSecRwRtStFrwdBkwdPos_Val/1 -> Terminator_33/1
  PA_KeSMSw6sVIPSecRwRtStFrwdBkwdPosMax_Val/1 -> Terminator_34/1
  PA_KeSMSw6sVIPSecRwRtStFrwdBkwdPosMin_Val/1 -> Terminator_35/1
  PA_KeSMSw6sVIPSecRwRtStFrwdBkwdPos_Val/1 -> Terminator_36/1
  PA_KeSMSwAcsEntrySecRwRtStFrwdBkwdPosMax_Val/1 -> Terminator_37/1
  PA_KeSMSwAcsEntrySecRwRtStFrwdBkwdPosMin_Val/1 -> Terminator_38/1
  PA_KeSMSwAcsEntrySecRwRtStFrwdBkwdPos_Val/1 -> Terminator_39/1
  PA_KeSMSwAcsExtSecRwRtStFrwdBkwdPosMax_Val/1 -> Terminator_40/1
  PA_KeSMSwAcsExtSecRwRtStFrwdBkwdPosMin_Val/1 -> Terminator_41/1
  PA_KeSMSwAcsExtSecRwRtStFrwdBkwdPos_Val/1 -> Terminator_42/1
  PA_KeSMSwFamilyMdSecRwRtStFrwdBkwdPosMax_Val/1 -> Terminator_43/1
  PA_KeSMSwFamilyMdSecRwRtStFrwdBkwdPosMin_Val/1 -> Terminator_44/1
  PA_KeSMSwFamilyMdSecRwRtStFrwdBkwdPos_Val/1 -> Terminator_45/1
  PA_KeSMSwFamilyRMdSecRwRtStFrwdBkwdPosMax_Val/1 -> Terminator_46/1
  PA_KeSMSwFamilyRMdSecRwRtStFrwdBkwdPosMin_Val/1 -> Terminator_47/1
  PA_KeSMSwFamilyRMdSecRwRtStFrwdBkwdPos_Val/1 -> Terminator_48/1
  PA_KeSMSwVIPSecRwRtStFrwdBkwdPosMax_Val/1 -> Terminator_49/1
  PA_KeSMSwVIPSecRwRtStFrwdBkwdPosMin_Val/1 -> Terminator_50/1
  PA_KeSMSwVIPSecRwRtStFrwdBkwdPos_Val/1 -> Terminator_51/1
  PA_KeSMSwAcsMd8SecRwRtStFrwdBkwdPosMax_Val/1 -> Terminator_52/1
  PA_KeSMSwAcsMd8SecRwRtStFrwdBkwdPosMin_Val/1 -> Terminator_53/1
  PA_KeSMSwAcsMd8SecRwRtStFrwdBkwdPos_Val/1 -> Terminator_54/1
  PA_KeSMSwAcsMd9SecRwRtStFrwdBkwdPosMax_Val/1 -> Terminator_55/1
  PA_KeSMSwAcsMd9SecRwRtStFrwdBkwdPosMin_Val/1 -> Terminator_56/1
  PA_KeSMSwAcsMd9SecRwRtStFrwdBkwdPos_Val/1 -> Terminator_57/1

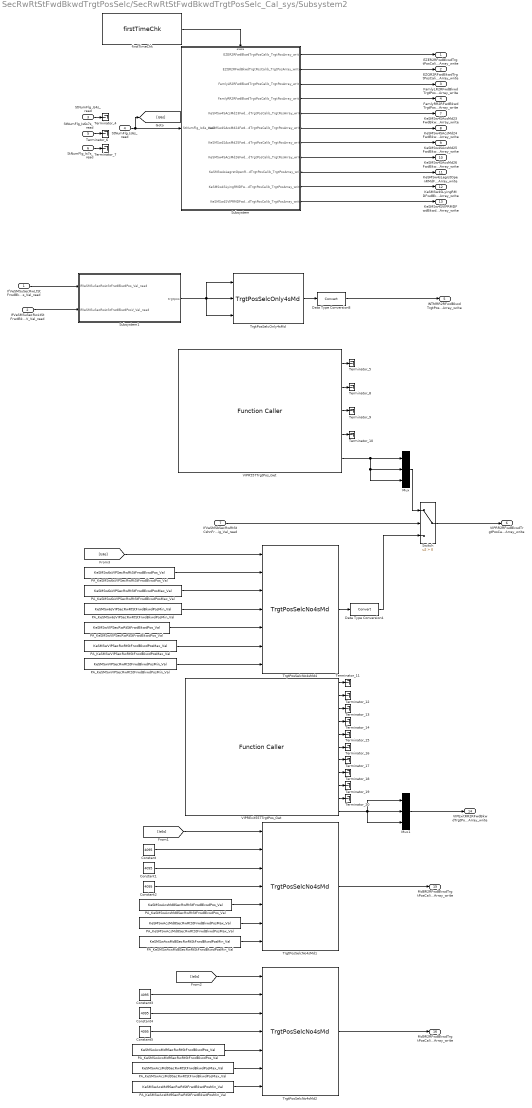
== system SecRwRtStFwdBkwdTrgtPosSelc/SecRwRtStFwdBkwdTrgtPosSelc_Cal_sys/Subsystem2 ==
  IfVeSMSuSecRwLtStFrwdBkwdPos_Val_read : Inport
  IfVeSMSuSecRwLtStFrwdBkwdPosV_Val_read : Inport  Port=2
  StNumFlg_Is4s_read : Inport  Port=3
  StNumFlg_Is6s_read : Inport  Port=4
  StNumFlg_Is6s7s_read : Inport  Port=5
  StNumFlg_Is7s_read : Inport  Port=6
  IfVeSMSbSecRwRtStCshnFrntUpwdDnwdMovConfig_Val_read : Inport  Port=7
  Constant{,1..5} (6 alike) : Constant  Value=4095  OutDataTypeStr=uint16
  Data Type Conversion4 : DataTypeConversion
  Data Type Conversion8 : DataTypeConversion
  Mux : Mux  Inputs=3
  Mux1 : Mux  Inputs=3
  PA_KeSMSw6sVIPSecRwRtStFrwdBkwdPosMax_Val : Constant  Value=KeSMSw6sVIPSecRwRtStFrwdBkwdPosMax_Val
  PA_KeSMSw6sVIPSecRwRtStFrwdBkwdPosMin_Val : Constant  Value=KeSMSw6sVIPSecRwRtStFrwdBkwdPosMin_Val
  PA_KeSMSw6sVIPSecRwRtStFrwdBkwdPos_Val : Constant  Value=KeSMSw6sVIPSecRwRtStFrwdBkwdPos_Val
  PA_KeSMSwAcsMd8SecRwRtStFrwdBkwdPosMax_Val : Constant  Value=KeSMSwAcsMd8SecRwRtStFrwdBkwdPosMax_Val
  PA_KeSMSwAcsMd8SecRwRtStFrwdBkwdPosMin_Val : Constant  Value=KeSMSwAcsMd8SecRwRtStFrwdBkwdPosMin_Val
  PA_KeSMSwAcsMd8SecRwRtStFrwdBkwdPos_Val : Constant  Value=KeSMSwAcsMd8SecRwRtStFrwdBkwdPos_Val
  PA_KeSMSwAcsMd9SecRwRtStFrwdBkwdPosMax_Val : Constant  Value=KeSMSwAcsMd9SecRwRtStFrwdBkwdPosMax_Val
  PA_KeSMSwAcsMd9SecRwRtStFrwdBkwdPosMin_Val : Constant  Value=KeSMSwAcsMd9SecRwRtStFrwdBkwdPosMin_Val
  PA_KeSMSwAcsMd9SecRwRtStFrwdBkwdPos_Val : Constant  Value=KeSMSwAcsMd9SecRwRtStFrwdBkwdPos_Val
  PA_KeSMSwVIPSecRwRtStFrwdBkwdPosMax_Val : Constant  Value=KeSMSwVIPSecRwRtStFrwdBkwdPosMax_Val
  PA_KeSMSwVIPSecRwRtStFrwdBkwdPosMin_Val : Constant  Value=KeSMSwVIPSecRwRtStFrwdBkwdPosMin_Val
  PA_KeSMSwVIPSecRwRtStFrwdBkwdPos_Val : Constant  Value=KeSMSwVIPSecRwRtStFrwdBkwdPos_Val
  Subsystem : Subsystem
  Subsystem1 : Subsystem
  Switch : Switch  Criteria=u2 > Threshold
  Terminator_{4..20} (17 alike) : Terminator
  TrgtPosSelcNo4sMd1 : TrgtPosSelcLib/TrgtPosSelcNo4sMd  SystemSampleTime=-1
  TrgtPosSelcNo4sMd2 : TrgtPosSelcLib/TrgtPosSelcNo4sMd  SystemSampleTime=-1
  TrgtPosSelcNo4sMd4 : TrgtPosSelcLib/TrgtPosSelcNo4sMd  SystemSampleTime=-1
  TrgtPosSelcOnly4sMd : TrgtPosSelcLib/TrgtPosSelcOnly4sMd  SystemSampleTime=-1
  VIPR557TrgtPos_Get : FunctionCaller  FunctionPrototype=[SecRwLtStBkReclnTrgtPos,SecRwLtStZeroTrgtPos,SecRwLtStLgrstUpwdDnwdTrgtPos,SecRwLtStLgrstInwdOtwdTrgtPos,SecRwLtStFwdBkwdTrgtPos] = VIPR557TrgtPos_Get()  OutputArgumentSpecifications=uint16(1), uint16(1), uint16(1), uint16(1), uint16(1)
  VIPRExit557TrgtPos_Get : FunctionCaller  FunctionPrototype=[SecRwRtStBkReclnTrgtPos,SecRwRtStZeroTrgtPos,SecRwRtStLgrstUpwdDnwdTrgtPos,SecRwRtStLgrstInwdOtwdTrgtPos,ThdRwLtStBkReclnTrgtPos,ThdRwLtStFwdBkwdTrgtPos,ThdRwRtStBkReclnTrgtPos,ThdRwRtStFwdBkwdTrgtPos,PassStBkReclnTrgtPos,PassStFwdBkwdTrgtPos,SecRwRtStFwdBkwdTrgtPos] = VIPRExit557TrgtPos_Get()  OutputArgumentSpecifications=uint16(1), uint16(1), uint16(1), uint16(1), uint16(1), uint16(1), uint16(1), uint16(1), uint16(1), uint16(1), uint16(1)
  firstTimeChk : TrgtPosSelcLib/firstTimeChk  SystemSampleTime=-1
  EZER2RFwdBkwdTrgtPosCalib_TrgtPosArray_write : Outport
      settings: EnsureOutportIsVirtual=on
  EZQR2RFwdBkwdTrgtPosCalib_TrgtPosArray_write : Outport  Port=2
      settings: EnsureOutportIsVirtual=on
  FamlyLR2RFwdBkwdTrgtPosCalib_TrgtPosArray_write : Outport  Port=3
      settings: EnsureOutportIsVirtual=on
  FamlyRR2RFwdBkwdTrgtPosCalib_TrgtPosArray_write : Outport  Port=4
      settings: EnsureOutportIsVirtual=on
  INTMRR2RFwdBkwdTrgtPosCalib_TrgtPosArray_write : Outport  Port=5
      settings: EnsureOutportIsVirtual=on
  VIPRR2RFwdBkwdTrgtPosCalib_TrgtPosArray_write : Outport  Port=6
      settings: EnsureOutportIsVirtual=on
  KeSMSw4SAcsMd23FwdBkwdTrgtPosCalib_TrgtPosArray_write : Outport  Port=7
      settings: EnsureOutportIsVirtual=on
  KeSMSw4SAcsMd24FwdBkwdTrgtPosCalib_TrgtPosArray_write : Outport  Port=8
      settings: EnsureOutportIsVirtual=on
  KeSMSw4SAcsMd25FwdBkwdTrgtPosCalib_TrgtPosArray_write : Outport  Port=9
      settings: EnsureOutportIsVirtual=on
  KeSMSw4SAcsMd26FwdBkwdTrgtPosCalib_TrgtPosArray_write : Outport  Port=10
      settings: EnsureOutportIsVirtual=on
  KeSMSw4sLegrstOpenRMdFwdBkwdTrgtPosCalib_TrgtPosArray_write : Outport  Port=11
      settings: EnsureOutportIsVirtual=on
  KeSMSw4SLyingRMDFwdBkwdTrgtPosCalib_TrgtPosArray_write : Outport  Port=12
      settings: EnsureOutportIsVirtual=on
  KeSMSw4SVIPRMDFwdBkwdTrgtPosCalib_TrgtPosArray_write : Outport  Port=13
      settings: EnsureOutportIsVirtual=on
  VIPExitRR2RFwdBkwdTrgtPosCalib_TrgtPosArray_write : Outport  Port=14
      settings: EnsureOutportIsVirtual=on
  Md8R2RFwdBkwdTrgtPosCalib_TrgtPosArray_write : Outport  Port=15
      settings: EnsureOutportIsVirtual=on
  Md9R2RFwdBkwdTrgtPosCalib_TrgtPosArray_write : Outport  Port=16
      settings: EnsureOutportIsVirtual=on
  wires:
  firstTimeChk/1 -> Subsystem/Enable
  StNumFlg_Is4s_read/1 -> Terminator_4/1
  Subsystem/4(FamlyRR2RFwdBkwdTrgtPosCalib_TrgtPosArray_write) -> FamlyRR2RFwdBkwdTrgtPosCalib_TrgtPosArray_write/1
  TrgtPosSelcOnly4sMd/1 -> Data Type Conversion8/1
  StNumFlg_Is6s_read/1 -> [Is6s], Subsystem/1(StNumFlg_Is6s_read)
  IfVeSMSuSecRwLtStFrwdBkwdPos_Val_read/1 -> Subsystem1/1(IfVeSMSuSecRwLtStFrwdBkwdPos_Val_read)
  IfVeSMSuSecRwLtStFrwdBkwdPosV_Val_read/1 -> Subsystem1/2(IfVeSMSuSecRwLtStFrwdBkwdPosV_Val_read)
  StNumFlg_Is7s_read/1 -> Terminator_7/1
  Subsystem/1(EZER2RFwdBkwdTrgtPosCalib_TrgtPosArray_write) -> EZER2RFwdBkwdTrgtPosCalib_TrgtPosArray_write/1
  Subsystem/2(EZQR2RFwdBkwdTrgtPosCalib_TrgtPosArray_write) -> EZQR2RFwdBkwdTrgtPosCalib_TrgtPosArray_write/1
  Subsystem/3(FamlyLR2RFwdBkwdTrgtPosCalib_TrgtPosArray_write) -> FamlyLR2RFwdBkwdTrgtPosCalib_TrgtPosArray_write/1
  StNumFlg_Is6s7s_read/1 -> Terminator_6/1
  Subsystem1/1(trgtpos) -> TrgtPosSelcOnly4sMd/1, TrgtPosSelcOnly4sMd/2, TrgtPosSelcOnly4sMd/3
  Subsystem/5(KeSMSw4SAcsMd23FwdBkwdTrgtPosCalib_TrgtPosArray_write) -> KeSMSw4SAcsMd23FwdBkwdTrgtPosCalib_TrgtPosArray_write/1
  Subsystem/6(KeSMSw4SAcsMd24FwdBkwdTrgtPosCalib_TrgtPosArray_write) -> KeSMSw4SAcsMd24FwdBkwdTrgtPosCalib_TrgtPosArray_write/1
  Subsystem/7(KeSMSw4SAcsMd25FwdBkwdTrgtPosCalib_TrgtPosArray_write) -> KeSMSw4SAcsMd25FwdBkwdTrgtPosCalib_TrgtPosArray_write/1
  Subsystem/8(KeSMSw4SAcsMd26FwdBkwdTrgtPosCalib_TrgtPosArray_write) -> KeSMSw4SAcsMd26FwdBkwdTrgtPosCalib_TrgtPosArray_write/1
  Data Type Conversion8/1 -> INTMRR2RFwdBkwdTrgtPosCalib_TrgtPosArray_write/1
  Subsystem/9(KeSMSw4sLegrstOpenRMdFwdBkwdTrgtPosCalib_TrgtPosArray_write) -> KeSMSw4sLegrstOpenRMdFwdBkwdTrgtPosCalib_TrgtPosArray_write/1
  Subsystem/10(KeSMSw4SLyingRMDFwdBkwdTrgtPosCalib_TrgtPosArray_write) -> KeSMSw4SLyingRMDFwdBkwdTrgtPosCalib_TrgtPosArray_write/1
  Subsystem/11(KeSMSw4SVIPRMDFwdBkwdTrgtPosCalib_TrgtPosArray_write) -> KeSMSw4SVIPRMDFwdBkwdTrgtPosCalib_TrgtPosArray_write/1
  IfVeSMSbSecRwRtStCshnFrntUpwdDnwdMovConfig_Val_read/1 -> Switch/2
  PA_KeSMSw6sVIPSecRwRtStFrwdBkwdPos_Val/1 -> TrgtPosSelcNo4sMd4/2
  [Is6s] -> TrgtPosSelcNo4sMd4/1
  PA_KeSMSwVIPSecRwRtStFrwdBkwdPosMax_Val/1 -> TrgtPosSelcNo4sMd4/6
  PA_KeSMSwVIPSecRwRtStFrwdBkwdPos_Val/1 -> TrgtPosSelcNo4sMd4/5
  PA_KeSMSw6sVIPSecRwRtStFrwdBkwdPosMax_Val/1 -> TrgtPosSelcNo4sMd4/3
  PA_KeSMSwVIPSecRwRtStFrwdBkwdPosMin_Val/1 -> TrgtPosSelcNo4sMd4/7
  TrgtPosSelcNo4sMd4/1 -> Data Type Conversion4/1
  PA_KeSMSw6sVIPSecRwRtStFrwdBkwdPosMin_Val/1 -> TrgtPosSelcNo4sMd4/4
  Data Type Conversion4/1 -> Switch/3
  Switch/1 -> VIPRR2RFwdBkwdTrgtPosCalib_TrgtPosArray_write/1
  VIPR557TrgtPos_Get/1 -> Terminator_5/1
  VIPR557TrgtPos_Get/2 -> Terminator_8/1
  VIPR557TrgtPos_Get/3 -> Terminator_9/1
  VIPR557TrgtPos_Get/4 -> Terminator_10/1
  Mux/1 -> Switch/1
  VIPR557TrgtPos_Get/5 -> Mux/3, Mux/2, Mux/1
  Mux1/1 -> VIPExitRR2RFwdBkwdTrgtPosCalib_TrgtPosArray_write/1
  VIPRExit557TrgtPos_Get/11 -> Mux1/3, Mux1/1, Mux1/2
  VIPRExit557TrgtPos_Get/1 -> Terminator_11/1
  VIPRExit557TrgtPos_Get/2 -> Terminator_12/1
  VIPRExit557TrgtPos_Get/3 -> Terminator_13/1
  VIPRExit557TrgtPos_Get/4 -> Terminator_14/1
  VIPRExit557TrgtPos_Get/5 -> Terminator_15/1
  VIPRExit557TrgtPos_Get/6 -> Terminator_16/1
  VIPRExit557TrgtPos_Get/7 -> Terminator_17/1
  VIPRExit557TrgtPos_Get/8 -> Terminator_18/1
  VIPRExit557TrgtPos_Get/9 -> Terminator_19/1
  VIPRExit557TrgtPos_Get/10 -> Terminator_20/1
  [Is6s] -> TrgtPosSelcNo4sMd1/1
  [Is6s] -> TrgtPosSelcNo4sMd2/1
  PA_KeSMSwAcsMd8SecRwRtStFrwdBkwdPos_Val/1 -> TrgtPosSelcNo4sMd1/5
  PA_KeSMSwAcsMd8SecRwRtStFrwdBkwdPosMax_Val/1 -> TrgtPosSelcNo4sMd1/6
  PA_KeSMSwAcsMd8SecRwRtStFrwdBkwdPosMin_Val/1 -> TrgtPosSelcNo4sMd1/7
  PA_KeSMSwAcsMd9SecRwRtStFrwdBkwdPos_Val/1 -> TrgtPosSelcNo4sMd2/5
  PA_KeSMSwAcsMd9SecRwRtStFrwdBkwdPosMax_Val/1 -> TrgtPosSelcNo4sMd2/6
  PA_KeSMSwAcsMd9SecRwRtStFrwdBkwdPosMin_Val/1 -> TrgtPosSelcNo4sMd2/7
  TrgtPosSelcNo4sMd1/1 -> Md8R2RFwdBkwdTrgtPosCalib_TrgtPosArray_write/1
  TrgtPosSelcNo4sMd2/1 -> Md9R2RFwdBkwdTrgtPosCalib_TrgtPosArray_write/1
  Constant/1 -> TrgtPosSelcNo4sMd1/2
  Constant1/1 -> TrgtPosSelcNo4sMd1/3
  Constant2/1 -> TrgtPosSelcNo4sMd1/4
  Constant3/1 -> TrgtPosSelcNo4sMd2/2
  Constant4/1 -> TrgtPosSelcNo4sMd2/3
  Constant5/1 -> TrgtPosSelcNo4sMd2/4

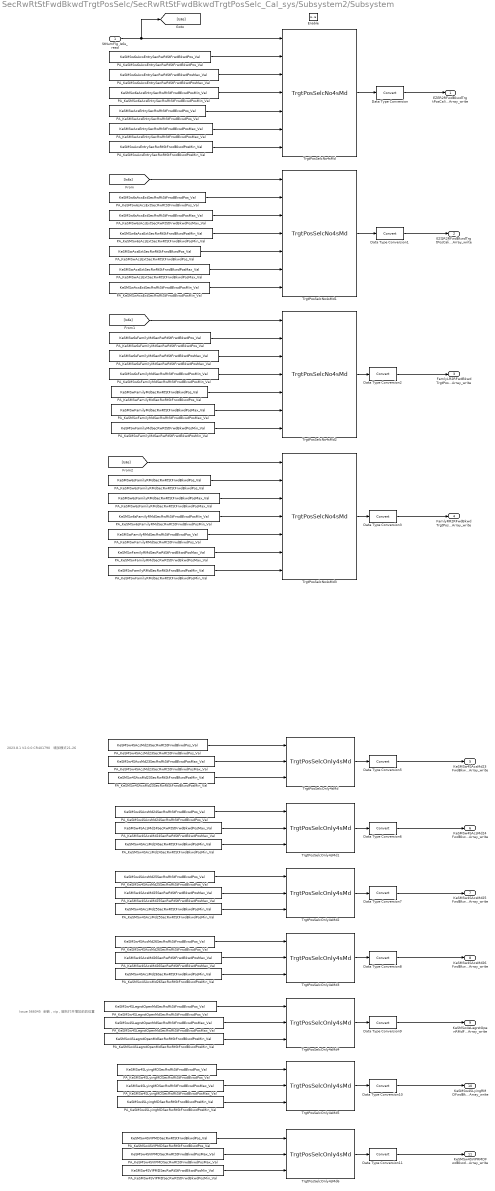
== system SecRwRtStFwdBkwdTrgtPosSelc/SecRwRtStFwdBkwdTrgtPosSelc_Cal_sys/Subsystem2/Subsystem ==
  note: Issue 566045 全躺，vip，腿托打开增加前后位置
  note: 2023.8.1 V2.0.0 CR401790 增加模式21-26
  StNumFlg_Is6s_read : Inport
  Enable : EnablePort
  Data Type Conversion{,1..3,5..11} (11 alike) : DataTypeConversion
  PA_KeSMSw4SAcsMd23SecRwRtStFrwdBkwdPosMax_Val : Constant  Value=KeSMSw4SAcsMd23SecRwRtStFrwdBkwdPosMax_Val
  PA_KeSMSw4SAcsMd23SecRwRtStFrwdBkwdPosMin_Val : Constant  Value=KeSMSw4SAcsMd23SecRwRtStFrwdBkwdPosMin_Val
  PA_KeSMSw4SAcsMd23SecRwRtStFrwdBkwdPos_Val : Constant  Value=KeSMSw4SAcsMd23SecRwRtStFrwdBkwdPos_Val
  PA_KeSMSw4SAcsMd24SecRwRtStFrwdBkwdPosMax_Val : Constant  Value=KeSMSw4SAcsMd24SecRwRtStFrwdBkwdPosMax_Val
  PA_KeSMSw4SAcsMd24SecRwRtStFrwdBkwdPosMin_Val : Constant  Value=KeSMSw4SAcsMd24SecRwRtStFrwdBkwdPosMin_Val
  PA_KeSMSw4SAcsMd24SecRwRtStFrwdBkwdPos_Val : Constant  Value=KeSMSw4SAcsMd24SecRwRtStFrwdBkwdPos_Val
  PA_KeSMSw4SAcsMd25SecRwRtStFrwdBkwdPosMax_Val : Constant  Value=KeSMSw4SAcsMd25SecRwRtStFrwdBkwdPosMax_Val
  PA_KeSMSw4SAcsMd25SecRwRtStFrwdBkwdPosMin_Val : Constant  Value=KeSMSw4SAcsMd25SecRwRtStFrwdBkwdPosMin_Val
  PA_KeSMSw4SAcsMd25SecRwRtStFrwdBkwdPos_Val : Constant  Value=KeSMSw4SAcsMd25SecRwRtStFrwdBkwdPos_Val
  PA_KeSMSw4SAcsMd26SecRwRtStFrwdBkwdPosMax_Val : Constant  Value=KeSMSw4SAcsMd26SecRwRtStFrwdBkwdPosMax_Val
  PA_KeSMSw4SAcsMd26SecRwRtStFrwdBkwdPosMin_Val : Constant  Value=KeSMSw4SAcsMd26SecRwRtStFrwdBkwdPosMin_Val
  PA_KeSMSw4SAcsMd26SecRwRtStFrwdBkwdPos_Val : Constant  Value=KeSMSw4SAcsMd26SecRwRtStFrwdBkwdPos_Val
  PA_KeSMSw4SLegrstOpenMdSecRwRtStFrwdBkwdPosMax_Val : Constant  Value=KeSMSw4SLegrstOpenMdSecRwRtStFrwdBkwdPosMax_Val
  PA_KeSMSw4SLegrstOpenMdSecRwRtStFrwdBkwdPosMin_Val : Constant  Value=KeSMSw4SLegrstOpenMdSecRwRtStFrwdBkwdPosMin_Val
  PA_KeSMSw4SLegrstOpenMdSecRwRtStFrwdBkwdPos_Val : Constant  Value=KeSMSw4SLegrstOpenMdSecRwRtStFrwdBkwdPos_Val
  PA_KeSMSw4SLyingMDSecRwRtStFrwdBkwdPosMax_Val : Constant  Value=KeSMSw4SLyingMDSecRwRtStFrwdBkwdPosMax_Val
  PA_KeSMSw4SLyingMDSecRwRtStFrwdBkwdPosMin_Val : Constant  Value=KeSMSw4SLyingMDSecRwRtStFrwdBkwdPosMin_Val
  PA_KeSMSw4SLyingMDSecRwRtStFrwdBkwdPos_Val : Constant  Value=KeSMSw4SLyingMDSecRwRtStFrwdBkwdPos_Val
  PA_KeSMSw4SVIPMDSecRwRtStFrwdBkwdPosMax_Val : Constant  Value=KeSMSw4SVIPMDSecRwRtStFrwdBkwdPosMax_Val
  PA_KeSMSw4SVIPMDSecRwRtStFrwdBkwdPosMin_Val : Constant  Value=KeSMSw4SVIPMDSecRwRtStFrwdBkwdPosMin_Val
  PA_KeSMSw4SVIPMDSecRwRtStFrwdBkwdPos_Val : Constant  Value=KeSMSw4SVIPMDSecRwRtStFrwdBkwdPos_Val
  PA_KeSMSw6sAcsEntrySecRwRtStFrwdBkwdPosMax_Val : Constant  Value=KeSMSw6sAcsEntrySecRwRtStFrwdBkwdPosMax_Val
  PA_KeSMSw6sAcsEntrySecRwRtStFrwdBkwdPosMin_Val : Constant  Value=KeSMSw6sAcsEntrySecRwRtStFrwdBkwdPosMin_Val
  PA_KeSMSw6sAcsEntrySecRwRtStFrwdBkwdPos_Val : Constant  Value=KeSMSw6sAcsEntrySecRwRtStFrwdBkwdPos_Val
  PA_KeSMSw6sAcsExtSecRwRtStFrwdBkwdPosMax_Val : Constant  Value=KeSMSw6sAcsExtSecRwRtStFrwdBkwdPosMax_Val
  PA_KeSMSw6sAcsExtSecRwRtStFrwdBkwdPosMin_Val : Constant  Value=KeSMSw6sAcsExtSecRwRtStFrwdBkwdPosMin_Val
  PA_KeSMSw6sAcsExtSecRwRtStFrwdBkwdPos_Val : Constant  Value=KeSMSw6sAcsExtSecRwRtStFrwdBkwdPos_Val
  PA_KeSMSw6sFamilyMdSecRwRtStFrwdBkwdPosMax_Val : Constant  Value=KeSMSw6sFamilyMdSecRwRtStFrwdBkwdPosMax_Val
  PA_KeSMSw6sFamilyMdSecRwRtStFrwdBkwdPosMin_Val : Constant  Value=KeSMSw6sFamilyMdSecRwRtStFrwdBkwdPosMin_Val
  PA_KeSMSw6sFamilyMdSecRwRtStFrwdBkwdPos_Val : Constant  Value=KeSMSw6sFamilyMdSecRwRtStFrwdBkwdPos_Val
  PA_KeSMSw6sFamilyRMdSecRwRtStFrwdBkwdPosMax_Val : Constant  Value=KeSMSw6sFamilyRMdSecRwRtStFrwdBkwdPosMax_Val
  PA_KeSMSw6sFamilyRMdSecRwRtStFrwdBkwdPosMin_Val : Constant  Value=KeSMSw6sFamilyRMdSecRwRtStFrwdBkwdPosMin_Val
  PA_KeSMSw6sFamilyRMdSecRwRtStFrwdBkwdPos_Val : Constant  Value=KeSMSw6sFamilyRMdSecRwRtStFrwdBkwdPos_Val
  PA_KeSMSwAcsEntrySecRwRtStFrwdBkwdPosMax_Val : Constant  Value=KeSMSwAcsEntrySecRwRtStFrwdBkwdPosMax_Val
  PA_KeSMSwAcsEntrySecRwRtStFrwdBkwdPosMin_Val : Constant  Value=KeSMSwAcsEntrySecRwRtStFrwdBkwdPosMin_Val
  PA_KeSMSwAcsEntrySecRwRtStFrwdBkwdPos_Val : Constant  Value=KeSMSwAcsEntrySecRwRtStFrwdBkwdPos_Val
  PA_KeSMSwAcsExtSecRwRtStFrwdBkwdPosMax_Val : Constant  Value=KeSMSwAcsExtSecRwRtStFrwdBkwdPosMax_Val
  PA_KeSMSwAcsExtSecRwRtStFrwdBkwdPosMin_Val : Constant  Value=KeSMSwAcsExtSecRwRtStFrwdBkwdPosMin_Val
  PA_KeSMSwAcsExtSecRwRtStFrwdBkwdPos_Val : Constant  Value=KeSMSwAcsExtSecRwRtStFrwdBkwdPos_Val
  PA_KeSMSwFamilyMdSecRwRtStFrwdBkwdPosMax_Val : Constant  Value=KeSMSwFamilyMdSecRwRtStFrwdBkwdPosMax_Val
  PA_KeSMSwFamilyMdSecRwRtStFrwdBkwdPosMin_Val : Constant  Value=KeSMSwFamilyMdSecRwRtStFrwdBkwdPosMin_Val
  PA_KeSMSwFamilyMdSecRwRtStFrwdBkwdPos_Val : Constant  Value=KeSMSwFamilyMdSecRwRtStFrwdBkwdPos_Val
  PA_KeSMSwFamilyRMdSecRwRtStFrwdBkwdPosMax_Val : Constant  Value=KeSMSwFamilyRMdSecRwRtStFrwdBkwdPosMax_Val
  PA_KeSMSwFamilyRMdSecRwRtStFrwdBkwdPosMin_Val : Constant  Value=KeSMSwFamilyRMdSecRwRtStFrwdBkwdPosMin_Val
  PA_KeSMSwFamilyRMdSecRwRtStFrwdBkwdPos_Val : Constant  Value=KeSMSwFamilyRMdSecRwRtStFrwdBkwdPos_Val
  TrgtPosSelcNo4sMd{,1..3} (4 alike) : TrgtPosSelcLib/TrgtPosSelcNo4sMd  SystemSampleTime=-1
  TrgtPosSelcOnly4sMd{,1..6} (7 alike) : TrgtPosSelcLib/TrgtPosSelcOnly4sMd  SystemSampleTime=-1
  EZER2RFwdBkwdTrgtPosCalib_TrgtPosArray_write : Outport
  EZQR2RFwdBkwdTrgtPosCalib_TrgtPosArray_write : Outport  Port=2
  FamlyLR2RFwdBkwdTrgtPosCalib_TrgtPosArray_write : Outport  Port=3
  FamlyRR2RFwdBkwdTrgtPosCalib_TrgtPosArray_write : Outport  Port=4
  KeSMSw4SAcsMd23FwdBkwdTrgtPosCalib_TrgtPosArray_write : Outport  Port=5
  KeSMSw4SAcsMd24FwdBkwdTrgtPosCalib_TrgtPosArray_write : Outport  Port=6
  KeSMSw4SAcsMd25FwdBkwdTrgtPosCalib_TrgtPosArray_write : Outport  Port=7
  KeSMSw4SAcsMd26FwdBkwdTrgtPosCalib_TrgtPosArray_write : Outport  Port=8
  KeSMSw4sLegrstOpenRMdFwdBkwdTrgtPosCalib_TrgtPosArray_write : Outport  Port=9
      settings: EnsureOutportIsVirtual=on
  KeSMSw4SLyingRMDFwdBkwdTrgtPosCalib_TrgtPosArray_write : Outport  Port=10
      settings: EnsureOutportIsVirtual=on
  KeSMSw4SVIPRMDFwdBkwdTrgtPosCalib_TrgtPosArray_write : Outport  Port=11
      settings: EnsureOutportIsVirtual=on
  wires:
  TrgtPosSelcNo4sMd2/1 -> Data Type Conversion2/1
  StNumFlg_Is6s_read/1 -> [Is6s], TrgtPosSelcNo4sMd/1
  TrgtPosSelcNo4sMd1/1 -> Data Type Conversion1/1
  TrgtPosSelcNo4sMd/1 -> Data Type Conversion/1
  TrgtPosSelcNo4sMd3/1 -> Data Type Conversion3/1
  PA_KeSMSw6sAcsEntrySecRwRtStFrwdBkwdPos_Val/1 -> TrgtPosSelcNo4sMd/2
  PA_KeSMSw6sAcsEntrySecRwRtStFrwdBkwdPosMax_Val/1 -> TrgtPosSelcNo4sMd/3
  PA_KeSMSw6sAcsEntrySecRwRtStFrwdBkwdPosMin_Val/1 -> TrgtPosSelcNo4sMd/4
  [Is6s] -> TrgtPosSelcNo4sMd1/1
  PA_KeSMSw6sAcsExtSecRwRtStFrwdBkwdPos_Val/1 -> TrgtPosSelcNo4sMd1/2
  PA_KeSMSw6sAcsExtSecRwRtStFrwdBkwdPosMax_Val/1 -> TrgtPosSelcNo4sMd1/3
  PA_KeSMSw6sAcsExtSecRwRtStFrwdBkwdPosMin_Val/1 -> TrgtPosSelcNo4sMd1/4
  [Is6s] -> TrgtPosSelcNo4sMd2/1
  PA_KeSMSw6sFamilyMdSecRwRtStFrwdBkwdPos_Val/1 -> TrgtPosSelcNo4sMd2/2
  PA_KeSMSw6sFamilyMdSecRwRtStFrwdBkwdPosMax_Val/1 -> TrgtPosSelcNo4sMd2/3
  PA_KeSMSw6sFamilyMdSecRwRtStFrwdBkwdPosMin_Val/1 -> TrgtPosSelcNo4sMd2/4
  [Is6s] -> TrgtPosSelcNo4sMd3/1
  PA_KeSMSw6sFamilyRMdSecRwRtStFrwdBkwdPos_Val/1 -> TrgtPosSelcNo4sMd3/2
  PA_KeSMSw6sFamilyRMdSecRwRtStFrwdBkwdPosMax_Val/1 -> TrgtPosSelcNo4sMd3/3
  PA_KeSMSw6sFamilyRMdSecRwRtStFrwdBkwdPosMin_Val/1 -> TrgtPosSelcNo4sMd3/4
  PA_KeSMSwAcsEntrySecRwRtStFrwdBkwdPosMax_Val/1 -> TrgtPosSelcNo4sMd/6
  PA_KeSMSwAcsEntrySecRwRtStFrwdBkwdPosMin_Val/1 -> TrgtPosSelcNo4sMd/7
  PA_KeSMSwAcsEntrySecRwRtStFrwdBkwdPos_Val/1 -> TrgtPosSelcNo4sMd/5
  PA_KeSMSwAcsExtSecRwRtStFrwdBkwdPosMax_Val/1 -> TrgtPosSelcNo4sMd1/6
  PA_KeSMSwAcsExtSecRwRtStFrwdBkwdPosMin_Val/1 -> TrgtPosSelcNo4sMd1/7
  PA_KeSMSwAcsExtSecRwRtStFrwdBkwdPos_Val/1 -> TrgtPosSelcNo4sMd1/5
  PA_KeSMSwFamilyMdSecRwRtStFrwdBkwdPosMax_Val/1 -> TrgtPosSelcNo4sMd2/6
  PA_KeSMSwFamilyMdSecRwRtStFrwdBkwdPosMin_Val/1 -> TrgtPosSelcNo4sMd2/7
  PA_KeSMSwFamilyMdSecRwRtStFrwdBkwdPos_Val/1 -> TrgtPosSelcNo4sMd2/5
  PA_KeSMSwFamilyRMdSecRwRtStFrwdBkwdPosMax_Val/1 -> TrgtPosSelcNo4sMd3/6
  PA_KeSMSwFamilyRMdSecRwRtStFrwdBkwdPos_Val/1 -> TrgtPosSelcNo4sMd3/5
  PA_KeSMSwFamilyRMdSecRwRtStFrwdBkwdPosMin_Val/1 -> TrgtPosSelcNo4sMd3/7
  TrgtPosSelcOnly4sMd3/1 -> Data Type Conversion8/1
  TrgtPosSelcOnly4sMd2/1 -> Data Type Conversion7/1
  TrgtPosSelcOnly4sMd1/1 -> Data Type Conversion6/1
  TrgtPosSelcOnly4sMd/1 -> Data Type Conversion5/1
  PA_KeSMSw4SAcsMd26SecRwRtStFrwdBkwdPosMax_Val/1 -> TrgtPosSelcOnly4sMd3/2
  PA_KeSMSw4SAcsMd26SecRwRtStFrwdBkwdPosMin_Val/1 -> TrgtPosSelcOnly4sMd3/3
  PA_KeSMSw4SAcsMd26SecRwRtStFrwdBkwdPos_Val/1 -> TrgtPosSelcOnly4sMd3/1
  PA_KeSMSw4SAcsMd25SecRwRtStFrwdBkwdPosMax_Val/1 -> TrgtPosSelcOnly4sMd2/2
  PA_KeSMSw4SAcsMd25SecRwRtStFrwdBkwdPosMin_Val/1 -> TrgtPosSelcOnly4sMd2/3
  PA_KeSMSw4SAcsMd25SecRwRtStFrwdBkwdPos_Val/1 -> TrgtPosSelcOnly4sMd2/1
  PA_KeSMSw4SAcsMd24SecRwRtStFrwdBkwdPosMax_Val/1 -> TrgtPosSelcOnly4sMd1/2
  PA_KeSMSw4SAcsMd24SecRwRtStFrwdBkwdPosMin_Val/1 -> TrgtPosSelcOnly4sMd1/3
  PA_KeSMSw4SAcsMd24SecRwRtStFrwdBkwdPos_Val/1 -> TrgtPosSelcOnly4sMd1/1
  PA_KeSMSw4SAcsMd23SecRwRtStFrwdBkwdPosMax_Val/1 -> TrgtPosSelcOnly4sMd/2
  PA_KeSMSw4SAcsMd23SecRwRtStFrwdBkwdPosMin_Val/1 -> TrgtPosSelcOnly4sMd/3
  PA_KeSMSw4SAcsMd23SecRwRtStFrwdBkwdPos_Val/1 -> TrgtPosSelcOnly4sMd/1
  Data Type Conversion/1 -> EZER2RFwdBkwdTrgtPosCalib_TrgtPosArray_write/1
  Data Type Conversion1/1 -> EZQR2RFwdBkwdTrgtPosCalib_TrgtPosArray_write/1
  Data Type Conversion2/1 -> FamlyLR2RFwdBkwdTrgtPosCalib_TrgtPosArray_write/1
  Data Type Conversion3/1 -> FamlyRR2RFwdBkwdTrgtPosCalib_TrgtPosArray_write/1
  Data Type Conversion5/1 -> KeSMSw4SAcsMd23FwdBkwdTrgtPosCalib_TrgtPosArray_write/1
  Data Type Conversion6/1 -> KeSMSw4SAcsMd24FwdBkwdTrgtPosCalib_TrgtPosArray_write/1
  Data Type Conversion7/1 -> KeSMSw4SAcsMd25FwdBkwdTrgtPosCalib_TrgtPosArray_write/1
  Data Type Conversion8/1 -> KeSMSw4SAcsMd26FwdBkwdTrgtPosCalib_TrgtPosArray_write/1
  PA_KeSMSw4SLegrstOpenMdSecRwRtStFrwdBkwdPos_Val/1 -> TrgtPosSelcOnly4sMd4/1
  PA_KeSMSw4SLegrstOpenMdSecRwRtStFrwdBkwdPosMin_Val/1 -> TrgtPosSelcOnly4sMd4/3
  PA_KeSMSw4SLegrstOpenMdSecRwRtStFrwdBkwdPosMax_Val/1 -> TrgtPosSelcOnly4sMd4/2
  TrgtPosSelcOnly4sMd4/1 -> Data Type Conversion9/1
  TrgtPosSelcOnly4sMd5/1 -> Data Type Conversion10/1
  PA_KeSMSw4SLyingMDSecRwRtStFrwdBkwdPosMax_Val/1 -> TrgtPosSelcOnly4sMd5/2
  PA_KeSMSw4SLyingMDSecRwRtStFrwdBkwdPosMin_Val/1 -> TrgtPosSelcOnly4sMd5/3
  PA_KeSMSw4SLyingMDSecRwRtStFrwdBkwdPos_Val/1 -> TrgtPosSelcOnly4sMd5/1
  PA_KeSMSw4SVIPMDSecRwRtStFrwdBkwdPos_Val/1 -> TrgtPosSelcOnly4sMd6/1
  PA_KeSMSw4SVIPMDSecRwRtStFrwdBkwdPosMin_Val/1 -> TrgtPosSelcOnly4sMd6/3
  PA_KeSMSw4SVIPMDSecRwRtStFrwdBkwdPosMax_Val/1 -> TrgtPosSelcOnly4sMd6/2
  TrgtPosSelcOnly4sMd6/1 -> Data Type Conversion11/1
  Data Type Conversion9/1 -> KeSMSw4sLegrstOpenRMdFwdBkwdTrgtPosCalib_TrgtPosArray_write/1
  Data Type Conversion11/1 -> KeSMSw4SVIPRMDFwdBkwdTrgtPosCalib_TrgtPosArray_write/1
  Data Type Conversion10/1 -> KeSMSw4SLyingRMDFwdBkwdTrgtPosCalib_TrgtPosArray_write/1

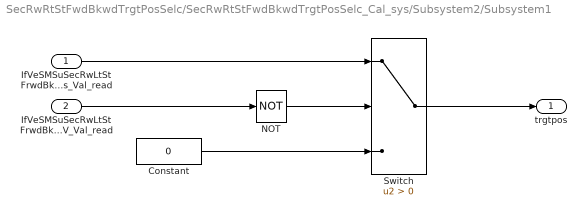
== system SecRwRtStFwdBkwdTrgtPosSelc/SecRwRtStFwdBkwdTrgtPosSelc_Cal_sys/Subsystem2/Subsystem1 ==
  IfVeSMSuSecRwLtStFrwdBkwdPos_Val_read : Inport
  IfVeSMSuSecRwLtStFrwdBkwdPosV_Val_read : Inport  Port=2
  Constant : Constant  Value=0  OutDataTypeStr=uint16
  NOT : Logic  Operator=NOT  AllPortsSameDT=off  OutDataTypeStr=boolean
  Switch : Switch  Criteria=u2 > Threshold
  trgtpos : Outport
  wires:
  IfVeSMSuSecRwLtStFrwdBkwdPos_Val_read/1 -> Switch/1
  IfVeSMSuSecRwLtStFrwdBkwdPosV_Val_read/1 -> NOT/1
  Constant/1 -> Switch/3
  NOT/1 -> Switch/2
  Switch/1 -> trgtpos/1
